simulink model "etc"  (R2020a)
settings: configuration reference "Configuration" (kept outside this file)
undefined symbols (not defined in the file): Cs, digital_range, direction_range_analog, duty_range_analog, J, Kd, Ks, sigbuilder_block, theta_eq, Ts, uint_range_10bit
libraries: adcUtils x2
settings Model: Creator=jrivitus  LastModifiedBy=Luiz
settings ConfigSetRef: SourceName=Configuration  SourceLocation=Base Workspace

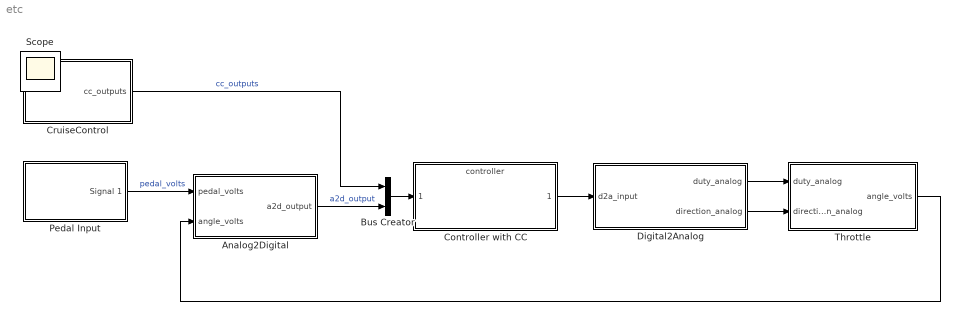
== system etc ==
  Analog2Digital : Subsystem
      settings: AttributesFormatString=(Hardware / software interface)  MinAlgLoopOccurrences=on
  Bus Creator : BusCreator  Inputs=2  OutDataTypeStr=Bus: ctrl_input_bus
  Controller with CC : ModelReference  ModelNameDialog=controller  SimulationMode=Normal  ModelReferenceVersion=1.146
      settings: AttributesFormatString=(Software)
  CruiseControl : Subsystem
      settings: MinAlgLoopOccurrences=on
  Digital2Analog : Subsystem
      settings: AttributesFormatString=(Software / hardware interface)  MinAlgLoopOccurrences=on
  Pedal Input : Subsystem  Tag=STV Subsys  LoadFcn=sigbuilder_block('load');  StartFcn=sigbuilder_block('start');  StopFcn=sigbuilder_block('stop');  ClipboardFcn=sigbuilder_block('clipboard');  mask(Sigbuilder block){tuvar=[0:10]}
      mask help: Sigbuilder GUI
      mask init:
      | if ~strcmp(get_param(bdroot(gcbh),'SimulationStatus'),'stopped') tuvar = sigbuilder_block('maskInit'); end
      settings: AttributesFormatString=0 - Pedal not pressed\n1 - Pedal fully pressed  CopyFcn=sigbuilder_block('copy');  DeleteFcn=sigbuilder_block('delete');  ModelCloseFcn=sigbuilder_block('modelClose');  PreSaveFcn=sigbuilder_block('preSave');  PauseFcn=sigbuilder_block('pause')  ContinueFcn=sigbuilder_block('continue')  NameChangeFcn=sigbuilder_block('namechange');  OpenFcn=sigbuilder_block('open',[44.069 297.31 550.552 397.862 ]);  CloseFcn=sigbuilder_block('close');
      mask Display: plot(0, 0, 100, 100,[2, 2, 32, 32, 2], [68, 8, 8, 68, 68],[32, 2], [38, 38], [32, 19, 2],[53, 60, 44], [32, 17, 17, 2],[16, 16, 31, 31]);txt = getActiveGroup(gcbh);text(2, 100, txt,'verticalAlignment', 'top');
  Throttle : Subsystem
      settings: AttributesFormatString=(Hardware - physical system)
  Scope : Scope
  wires:
  Analog2Digital/1(a2d_output) -> Bus Creator/2  "a2d_output"
  CruiseControl/1(cc_outputs) -> Bus Creator/1  "cc_outputs"
  Digital2Analog/1(duty_analog) -> Throttle/1(duty_analog)
  Digital2Analog/2(direction_analog) -> Throttle/2(direction_analog)
  Throttle/1(angle_volts) -> Analog2Digital/2(angle_volts)
  Pedal Input/1(Signal 1) -> Analog2Digital/1(pedal_volts)  "pedal_volts"
  Bus Creator/1 -> Controller with CC/1
  Controller with CC/1 -> Digital2Analog/1(d2a_input)

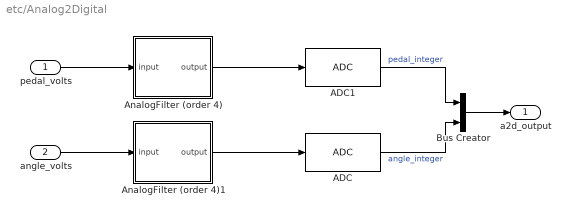
== system etc/Analog2Digital ==
  pedal_volts : Inport  OutDataTypeStr=double  PortDimensions=1  SampleTime=0
  angle_volts : Inport  Port=2  OutDataTypeStr=double  PortDimensions=1  SampleTime=0
  ADC : adcUtils/ADC  analog_range=angle_sensor_range  digital_range=uint_range_10bit  outputType=uint16  sampleRate=Ts
  ADC1 : adcUtils/ADC  analog_range=pedal_sensor_range  digital_range=uint_range_10bit  outputType=uint16  sampleRate=Ts
  AnalogFilter (order 4) : Subsystem  VariantControl=analogFilter==1
  AnalogFilter (order 4)1 : Subsystem  VariantControl=analogFilter==1
  Bus Creator : BusCreator  Inputs=2  OutDataTypeStr=Bus: a2d_output_bus
  a2d_output : Outport  OutDataTypeStr=Bus: a2d_output_bus  SampleTime=Ts  VectorParamsAs1DForOutWhenUnconnected=off
  wires:
  pedal_volts/1 -> AnalogFilter (order 4)/1(input)
  angle_volts/1 -> AnalogFilter (order 4)1/1(input)
  ADC1/1 -> Bus Creator/1  "pedal_integer"
  ADC/1 -> Bus Creator/2  "angle_integer"
  Bus Creator/1 -> a2d_output/1
  AnalogFilter (order 4)/1(output) -> ADC1/1
  AnalogFilter (order 4)1/1(output) -> ADC/1

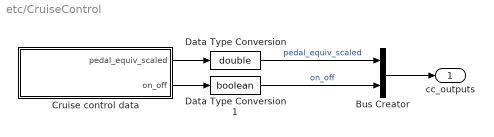
== system etc/CruiseControl ==
  Bus Creator : BusCreator  Inputs=2  OutDataTypeStr=Bus: cc_outputs_bus
  Cruise control data : Subsystem  Tag=STV Subsys  LoadFcn=sigbuilder_block('load');  StartFcn=sigbuilder_block('start');  StopFcn=sigbuilder_block('stop');  ClipboardFcn=sigbuilder_block('clipboard');  mask(Sigbuilder block){tuvar=[0:10]}
      mask help: Sigbuilder GUI
      mask init:
      | if ~strcmp(get_param(bdroot(gcbh),'SimulationStatus'),'stopped') tuvar = sigbuilder_block('maskInit'); end
      settings: CopyFcn=sigbuilder_block('copy');  DeleteFcn=sigbuilder_block('delete');  ModelCloseFcn=sigbuilder_block('modelClose');  PreSaveFcn=sigbuilder_block('preSave');  PauseFcn=sigbuilder_block('pause')  ContinueFcn=sigbuilder_block('continue')  NameChangeFcn=sigbuilder_block('namechange');  OpenFcn=sigbuilder_block('open',[44.069 296.69 550.552 398.483 ]);  CloseFcn=sigbuilder_block('close');
      mask Display: plot(0, 0, 100, 100,[2, 2, 32, 32, 2], [68, 8, 8, 68, 68],[32, 2], [38, 38], [32, 19, 2],[53, 60, 44], [32, 17, 17, 2],[16, 16, 31, 31]);txt = getActiveGroup(gcbh);text(2, 100, txt,'verticalAlignment', 'top');
  Data Type Conversion : DataTypeConversion  OutDataTypeStr=double  SampleTime=Ts
  Data Type Conversion1 : DataTypeConversion  OutDataTypeStr=boolean  SampleTime=Ts
  cc_outputs : Outport  OutDataTypeStr=Bus: cc_outputs_bus  SampleTime=Ts  VectorParamsAs1DForOutWhenUnconnected=off
  wires:
  Cruise control data/1(pedal_equiv_scaled) -> Data Type Conversion/1
  Cruise control data/2(on_off) -> Data Type Conversion1/1
  Data Type Conversion/1 -> Bus Creator/1  "pedal_equiv_scaled"
  Data Type Conversion1/1 -> Bus Creator/2  "on_off"
  Bus Creator/1 -> cc_outputs/1

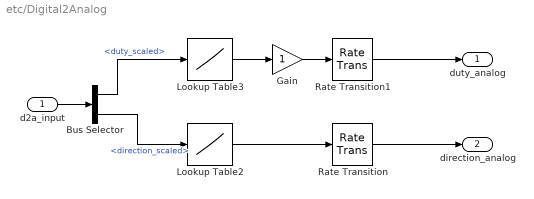
== system etc/Digital2Analog ==
  d2a_input : Inport  OutDataTypeStr=Bus: d2a_input_bus  PortDimensions=1  SampleTime=Ts
  Bus Selector : BusSelector  OutputSignals=duty_scaled,direction_scaled
  Gain : Gain
  Lookup Table2 : Lookup_n-D  NumberOfTableDimensions=1  BreakpointsForDimension1=digital_range  Table=direction_range_analog  ExtrapMethod=Clip  OutDataTypeStr=double  InputSameDT=on
      settings: AttributesFormatString=Output data type: %<OutDataTypeStr>
  Lookup Table3 : Lookup_n-D  NumberOfTableDimensions=1  BreakpointsForDimension1=uint_range_10bit  Table=duty_range_analog  ExtrapMethod=Clip  OutDataTypeStr=double  InputSameDT=on
      settings: AttributesFormatString=Output data type: %<OutDataTypeStr>
  Rate Transition : RateTransition  Integrity=off  OutPortSampleTime=0
  Rate Transition1 : RateTransition  Integrity=off  OutPortSampleTime=0
  duty_analog : Outport  OutDataTypeStr=double  PortDimensions=1  SampleTime=0  VectorParamsAs1DForOutWhenUnconnected=off
  direction_analog : Outport  Port=2  OutDataTypeStr=double  PortDimensions=1  SampleTime=0  VectorParamsAs1DForOutWhenUnconnected=off
  wires:
  Bus Selector/2 -> Lookup Table2/1  "<direction_scaled>"
  Bus Selector/1 -> Lookup Table3/1  "<duty_scaled>"
  Rate Transition/1 -> direction_analog/1
  Rate Transition1/1 -> duty_analog/1
  d2a_input/1 -> Bus Selector/1
  Gain/1 -> Rate Transition1/1
  Lookup Table3/1 -> Gain/1
  Lookup Table2/1 -> Rate Transition/1

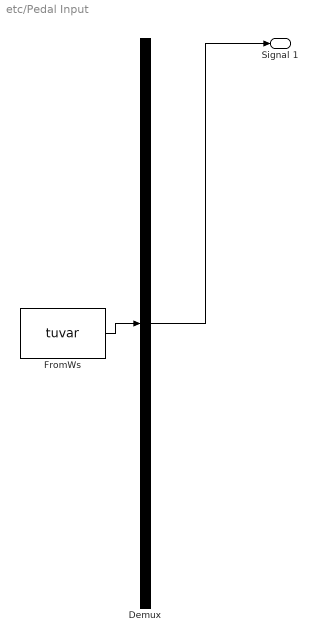
== system etc/Pedal Input ==
  Demux : Demux  Tag=STV Demux  Outputs=1
      settings: DisplayOption=none
  FromWs : FromWorkspace  Tag=STV FromWs  VariableName=tuvar
      SigBuilderData=|
      | common.afterFinalStr = 'Extrapolate'
      | common.sampleTime = 0
      | dataSet(1).timeRange = [0 10]
      | dataSet(1).name = 'Group 1'
      | dataSet(2).timeRange = [0 10]
      | dataSet(2).name = 'Group 2'
      | sbobj.Groups(1).Name = 'Group 1'
      | sbobj.Groups(1).Signals.Name = 'Signal 1'
      | sbobj.Groups(1).Signals.XData = [0 2 2 10]
      | sbobj.Groups(1).Signals.YData = [0 0 0.8 0.8]
      | sbobj.Groups(2).Name = 'Group 2'
      | sbobj.Groups(2).Signals.Name = 'Signal 1'
      | sbobj.Groups(2).Signals.XData = [0 2 2 6.58 6.58 10]
      | sbobj.Groups(2).Signals.YData = [0.586 0.586 0.267 0.267 0.0195 0.0195]
  Signal 1 : Outport  Tag=STV Outport  VectorParamsAs1DForOutWhenUnconnected=off
  wires:
  Demux/1 -> Signal 1/1
  FromWs/1 -> Demux/1

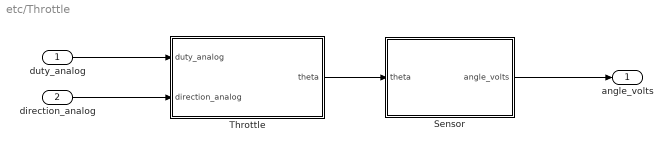
== system etc/Throttle ==
  duty_analog : Inport  OutDataTypeStr=double  PortDimensions=1  SampleTime=0
  direction_analog : Inport  Port=2  OutDataTypeStr=double  PortDimensions=1  SampleTime=0
  Sensor : Subsystem
  Throttle : Subsystem
  angle_volts : Outport  OutDataTypeStr=double  PortDimensions=1  SampleTime=0  VectorParamsAs1DForOutWhenUnconnected=off
  wires:
  duty_analog/1 -> Throttle/1(duty_analog)
  direction_analog/1 -> Throttle/2(direction_analog)
  Throttle/1(theta) -> Sensor/1(theta)
  Sensor/1(angle_volts) -> angle_volts/1

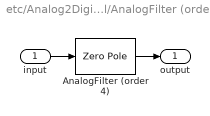
== system etc/Analog2Digital/AnalogFilter (order 4) ==
  input : Inport
  AnalogFilter (order 4) : ZeroPole  Zeros=[]  Poles=1.0e2*[-2.2739+0.6809i,-2.2739-0.6809i,-1.6518+2.0864i,-1.6518-2.0864i]  Gain=3.9899e9
  output : Outport  VectorParamsAs1DForOutWhenUnconnected=off
  wires:
  input/1 -> AnalogFilter (order 4)/1
  AnalogFilter (order 4)/1 -> output/1

== system etc/Analog2Digital/AnalogFilter (order 4)1 ==
  input : Inport
  AnalogFilter (order 4) : ZeroPole  Zeros=[]  Poles=1.0e2*[-2.2739+0.6809i,-2.2739-0.6809i,-1.6518+2.0864i,-1.6518-2.0864i]  Gain=3.9899e9
  output : Outport  VectorParamsAs1DForOutWhenUnconnected=off
  wires:
  AnalogFilter (order 4)/1 -> output/1
  input/1 -> AnalogFilter (order 4)/1

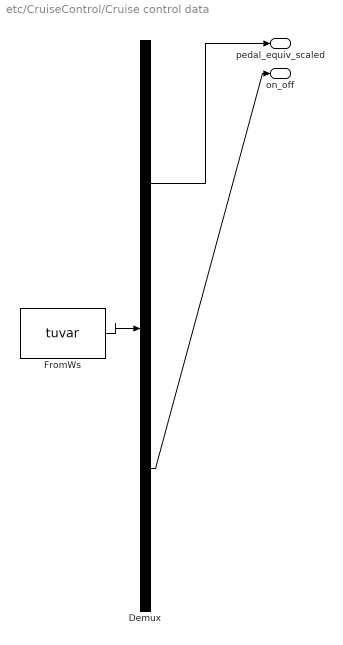
== system etc/CruiseControl/Cruise control data ==
  Demux : Demux  Tag=STV Demux  Outputs=2
      settings: DisplayOption=none
  FromWs : FromWorkspace  Tag=STV FromWs  VariableName=tuvar
      SigBuilderData=|
      | common.afterFinalStr = 'Extrapolate'
      | common.sampleTime = 0
      | dataSet.timeRange = [0 10]
      | dataSet.name = 'Group 1'
      | sbobj.Groups.Name = 'Group 1'
      | sbobj.Groups.Signals(1).Name = 'pedal_equiv_scaled'
      | sbobj.Groups.Signals(1).XData = [0 4 4 10]
      | sbobj.Groups.Signals(1).YData = [0 0 2.42 2.42]
      | sbobj.Groups.Signals(2).Name = 'on_off'
      | sbobj.Groups.Signals(2).XData = [0 4 4 10]
      | sbobj.Groups.Signals(2).YData = [0 0 1 1]
  pedal_equiv_scaled : Outport  Tag=STV Outport  VectorParamsAs1DForOutWhenUnconnected=off
  on_off : Outport  Tag=STV Outport  Port=2  VectorParamsAs1DForOutWhenUnconnected=off
  wires:
  FromWs/1 -> Demux/1
  Demux/1 -> pedal_equiv_scaled/1
  Demux/2 -> on_off/1

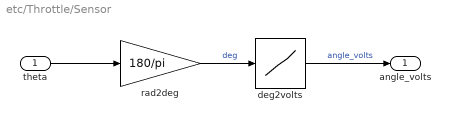
== system etc/Throttle/Sensor ==
  theta : Inport
  deg2volts : Lookup  InputValues=[0 90]  Table=[0.5 4.5]  LookUpMeth=Interpolation-Use End Values
  rad2deg : Gain  Gain=180/pi  SaturateOnIntegerOverflow=on  OutDataTypeStr=Inherit: Same as input  ParamDataTypeStr=Inherit: Same as input
  angle_volts : Outport  VectorParamsAs1DForOutWhenUnconnected=off
  wires:
  theta/1 -> rad2deg/1
  deg2volts/1 -> angle_volts/1  "angle_volts"
  rad2deg/1 -> deg2volts/1  "deg"

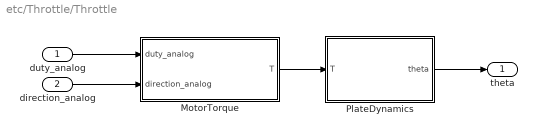
== system etc/Throttle/Throttle ==
  duty_analog : Inport
  direction_analog : Inport  Port=2
  MotorTorque : Subsystem
  PlateDynamics : Subsystem
  theta : Outport  VectorParamsAs1DForOutWhenUnconnected=off
  wires:
  MotorTorque/1(T) -> PlateDynamics/1(T)
  duty_analog/1 -> MotorTorque/1(duty_analog)
  direction_analog/1 -> MotorTorque/2(direction_analog)
  PlateDynamics/1(theta) -> theta/1

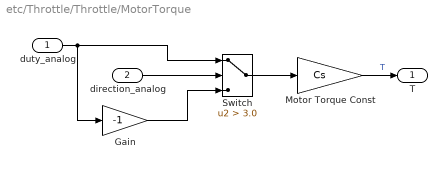
== system etc/Throttle/Throttle/MotorTorque ==
  duty_analog : Inport
  direction_analog : Inport  Port=2
  Gain : Gain  Gain=-1  SaturateOnIntegerOverflow=on  OutDataTypeStr=Inherit: Same as input  ParamDataTypeStr=Inherit: Same as input
  Motor Torque Const : Gain  Gain=Cs  SaturateOnIntegerOverflow=on  OutDataTypeStr=Inherit: Same as input  ParamDataTypeStr=Inherit: Same as input
  Switch : Switch  Criteria=u2 > Threshold  Threshold=3.0
  T : Outport  VectorParamsAs1DForOutWhenUnconnected=off
  wires:
  Switch/1 -> Motor Torque Const/1
  direction_analog/1 -> Switch/2
  duty_analog/1 -> Switch/1, Gain/1
  Gain/1 -> Switch/3
  Motor Torque Const/1 -> T/1  "T"

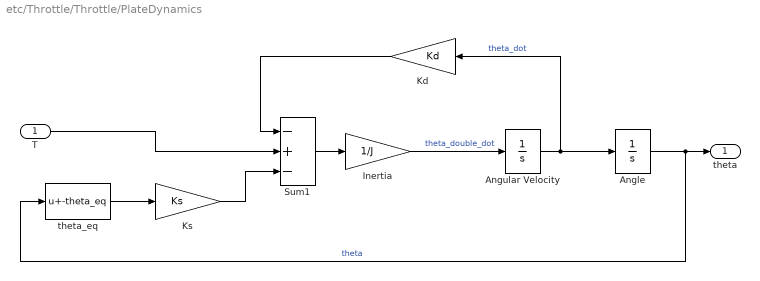
== system etc/Throttle/Throttle/PlateDynamics ==
  T : Inport
  Angle : Integrator  InitialCondition=theta_eq  LimitOutput=on  UpperSaturationLimit=pi/2  LowerSaturationLimit=0
      settings: AttributesFormatString=Initial condition: %<InitialCondition>\n%<LowerSaturationLimit> <= theta <= %<UpperSaturationLimit>
  Angular Velocity : Integrator
      settings: AttributesFormatString=Initial condition: %<InitialCondition>
  Inertia : Gain  Gain=1/J  SaturateOnIntegerOverflow=on  OutDataTypeStr=Inherit: Same as input  ParamDataTypeStr=Inherit: Same as input
  Kd : Gain  Gain=Kd  SaturateOnIntegerOverflow=on  OutDataTypeStr=Inherit: Same as input  ParamDataTypeStr=Inherit: Same as input
  Ks : Gain  Gain=Ks  SaturateOnIntegerOverflow=on  OutDataTypeStr=Inherit: Same as input  ParamDataTypeStr=Inherit: Same as input
  Sum1 : Sum  Inputs=-+-  SaturateOnIntegerOverflow=on
  theta_eq : Bias  Bias=-theta_eq
  theta : Outport  VectorParamsAs1DForOutWhenUnconnected=off
  wires:
  theta_eq/1 -> Ks/1
  Angle/1 -> theta/1, theta_eq/1  "theta"
  Angular Velocity/1 -> Angle/1, Kd/1  "theta_dot"
  Inertia/1 -> Angular Velocity/1  "theta_double_dot"
  Sum1/1 -> Inertia/1
  Kd/1 -> Sum1/1
  Ks/1 -> Sum1/3
  T/1 -> Sum1/2
